simulink model "bitwise"  (R2021a)
settings: Solver=FixedStepDiscrete  StartTime=0.0  StopTime=10.0  RelTol=1e-3  EnableMultiTasking=on
libraries: simulink x7
settings Model: Creator=omar  LastModifiedBy=omar
settings DataIOCC: ReturnWorkspaceOutputs=off
settings OptimizationCC: DefaultParameterBehavior=Inlined  InlineInvariantSignals=on  EnableMemcpy=off  LifeSpan=1  EfficientTunableParamExpr=on
settings DebuggingCC: UnderspecifiedInitializationDetection=Classic  MergeDetectMultiDrivingBlocksExec=none  SFMachineParentedDataDiag=warning  ArithmeticOperatorsInVariantConditions=warning
settings ModelReferenceCC: PropagateSignalLabelsOutOfModel=off
settings SFSimCC: MATLABDynamicMemAlloc=off  CustomCodeUndefinedFunction=UseInterfaceOnly
settings RTWCC: SystemTargetFile=ert.tlc  GenCodeOnly=on  TemplateMakefile=ert_default_tmf  GenerateReport=on  IncludeHyperlinkInReport=on  LaunchReport=on  GenerateTraceInfo=on  GenerateTraceReport=on  GenerateTraceReportSl=on  GenerateTraceReportSf=on  GenerateTraceReportEml=on
settings CodeAppCC: ForceParamTrailComments=on  IgnoreCustomStorageClasses=off  OperatorAnnotations=on  SimulinkDataObjDesc=on  SFDataObjDesc=on  MATLABFcnDesc=on  InsertBlockDesc=on  StateflowObjectComments=on  MATLABSourceComments=on
settings ERTTargetCC: MultiwordLength=2048  GenerateSampleERTMain=on  InlinedParameterPlacement=NonHierarchical  ERTCustomFileTemplate=example_file_process.tlc

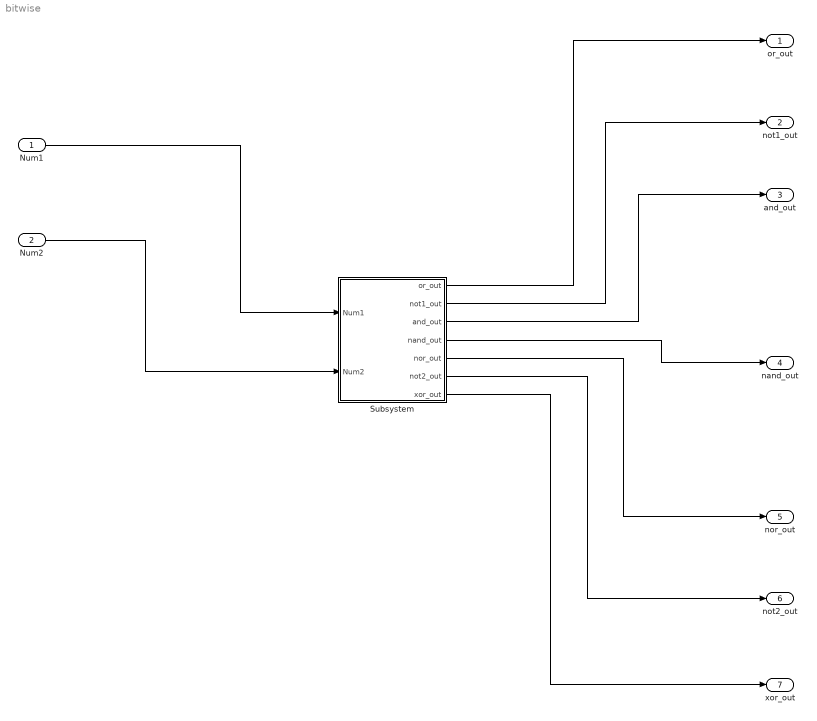
== system bitwise ==
  Num1 : Inport
  Num2 : Inport  Port=2
  Subsystem : Subsystem
  or_out : Outport
  not1_out : Outport  Port=2
  and_out : Outport  Port=3
  nand_out : Outport  Port=4
  nor_out : Outport  Port=5
  not2_out : Outport  Port=6
  xor_out : Outport  Port=7
  wires:
  Num1/1 -> Subsystem/1(Num1)
  Num2/1 -> Subsystem/2(Num2)
  Subsystem/1(or_out) -> or_out/1
  Subsystem/2(not1_out) -> not1_out/1
  Subsystem/3(and_out) -> and_out/1
  Subsystem/4(nand_out) -> nand_out/1
  Subsystem/5(nor_out) -> nor_out/1
  Subsystem/6(not2_out) -> not2_out/1
  Subsystem/7(xor_out) -> xor_out/1

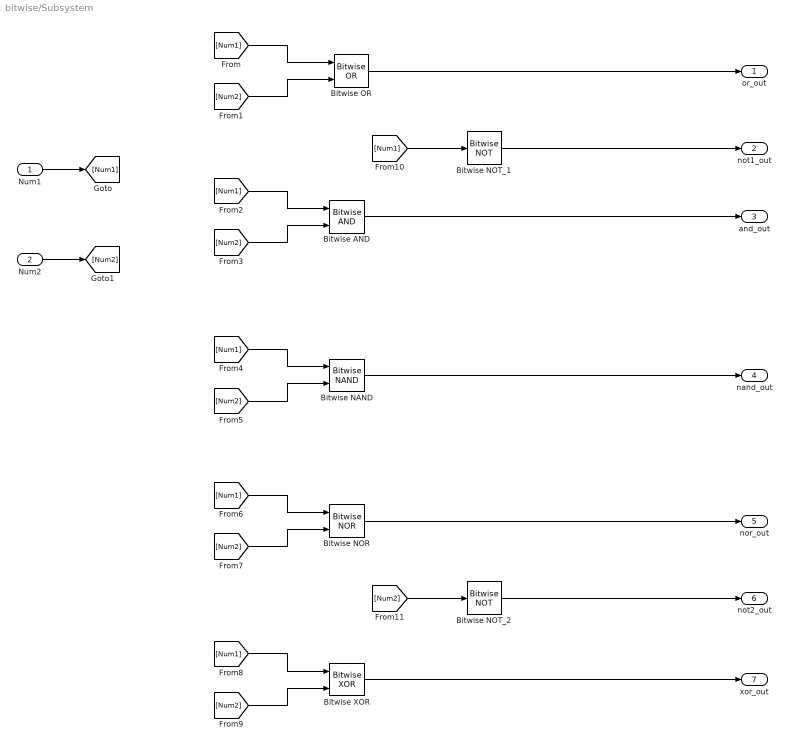
== system bitwise/Subsystem ==
  Num1 : Inport  OutDataTypeStr=uint32
  Num2 : Inport  Port=2  OutDataTypeStr=uint32
  Bitwise AND : simulink/Logic and Bit Operations/Bitwise Operator  logicop=AND  UseBitMask=off  NumInputPorts=2  BitMask=bin2dec('11011001')  BitMaskRealWorld=Stored Integer
  Bitwise NAND : simulink/Logic and Bit Operations/Bitwise Operator  logicop=NAND  UseBitMask=off  NumInputPorts=2  BitMask=bin2dec('11011001')  BitMaskRealWorld=Stored Integer
  Bitwise NOR : simulink/Logic and Bit Operations/Bitwise Operator  logicop=NOR  UseBitMask=off  NumInputPorts=2  BitMask=bin2dec('11011001')  BitMaskRealWorld=Stored Integer
  Bitwise NOT_1 : simulink/Logic and Bit Operations/Bitwise Operator  logicop=NOT  UseBitMask=off  BitMask=bin2dec('11011001')  BitMaskRealWorld=Stored Integer
  Bitwise NOT_2 : simulink/Logic and Bit Operations/Bitwise Operator  logicop=NOT  UseBitMask=off  BitMask=bin2dec('11011001')  BitMaskRealWorld=Stored Integer
  Bitwise OR : simulink/Logic and Bit Operations/Bitwise Operator  logicop=OR  UseBitMask=off  NumInputPorts=2  BitMask=bin2dec('11011001')  BitMaskRealWorld=Stored Integer
  Bitwise XOR : simulink/Logic and Bit Operations/Bitwise Operator  logicop=XOR  UseBitMask=off  NumInputPorts=2  BitMask=bin2dec('11011001')  BitMaskRealWorld=Stored Integer
  or_out : Outport
  not1_out : Outport  Port=2
  and_out : Outport  Port=3
  nand_out : Outport  Port=4
  nor_out : Outport  Port=5
  not2_out : Outport  Port=6
  xor_out : Outport  Port=7
  wires:
  [Num2] -> Bitwise NAND/2
  [Num1] -> Bitwise OR/1
  [Num1] -> Bitwise XOR/1
  Num1/1 -> [Num1]
  [Num1] -> Bitwise NAND/1
  [Num1] -> Bitwise NOT_1/1
  [Num1] -> Bitwise AND/1
  Bitwise XOR/1 -> xor_out/1
  Bitwise AND/1 -> and_out/1
  Num2/1 -> [Num2]
  [Num2] -> Bitwise XOR/2
  Bitwise NAND/1 -> nand_out/1
  [Num2] -> Bitwise NOT_2/1
  Bitwise NOT_2/1 -> not2_out/1
  Bitwise OR/1 -> or_out/1
  [Num2] -> Bitwise NOR/2
  [Num1] -> Bitwise NOR/1
  Bitwise NOT_1/1 -> not1_out/1
  Bitwise NOR/1 -> nor_out/1
  [Num2] -> Bitwise AND/2
  [Num2] -> Bitwise OR/2
